simulink model "Radiometer_System_Model"  (R2019b)
settings: Solver=FixedStepDiscrete  StartTime=0.0  StopTime=0.00011  FixedStep=1/2500e6  RelTol=1e-3  EnableMultiTasking=on
values from neighbouring files (symbols this model uses):
  ADC_Clock = 2500e6    (= 2500000000)    [RunMe.m]
  divisionConst = 50    [RunMe.m]
libraries: dspsrcs4 x2
settings Model: Creator=tmacleod  LastModifiedBy=ian
settings SolverCC: AutoInsertRateTranBlk=on
settings DataIOCC: LimitDataPoints=on  SaveFormat=Array  ReturnWorkspaceOutputs=off
settings OptimizationCC: LifeSpan=inf
settings DebuggingCC: SolverPrmCheckMsg=warning  SFUnexpectedBacktrackingDiag=warning  SFNoUnconditionalDefaultTransitionDiag=warning  SFExecutionAtInitializationDiag=none  ArithmeticOperatorsInVariantConditions=warning
settings HardwareCC: ProdBitPerPointer=32  ProdBitPerSizeT=32  ProdBitPerPtrDiffT=32  ProdLargestAtomicFloat=None  ProdIntDivRoundTo=Undefined  ProdEndianess=Unspecified  ProdWordSize=32  ProdHWDeviceType=32-bit Generic
settings ModelReferenceCC: PropagateSignalLabelsOutOfModel=off
settings SFSimCC: SimUseLocalCustomCode=off  CustomCodeUndefinedFunction=UseInterfaceOnly
settings RTWCC: RTWUseLocalCustomCode=off
settings CodeAppCC: StateflowObjectComments=on
settings GRTTargetCC: TargetLangStandard=C89/C90 (ANSI)  GeneratePreprocessorConditionals=Disable all
settings ConfigComp: CovMetricSettings=dw  CovHtmlReporting=on  CovSaveCumulativeToWorkspaceVar=on  CovSaveSingleToWorkspaceVar=on  CovExternalEMLEnable=off  CovSFcnEnable=off

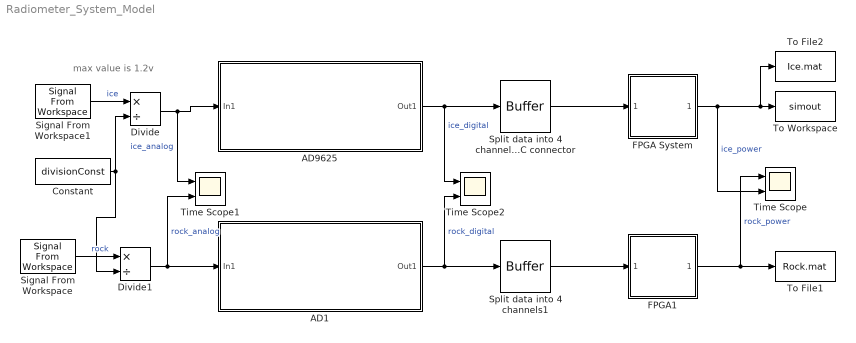
== system Radiometer_System_Model ==
  note: max value is 1.2v
  AD1 : Subsystem  mask{maskMode=ADC Only, maskDecimation=8, maskGain=0, maskNcoFreq=100e6, maskFclk=ADC_Clock, maskTessitura=147e6, maskExtJitter=60e-15, maskInputConfig=Absolute}
      mask prompts: maskMode "Mode of Operation"; maskDecimation "DDC Decimation"; maskGain "DDC Gain (dB)"; maskNcoFreq "NCO Frequency (Hz)"; maskFclk "Sampling Clock Frequency (Hz)"; maskTessitura "Mean Frequency (Hz)"; maskExtJitter "RMS Clock Jitter"; maskInputConfig "Input Configuration"
      mask init:
      | set_param([gcb '/AD9625 System Object'], 'Mode', maskMode);
      | set_param([gcb '/AD9625 System Object'], 'Decimation', maskDecimation);
      | set_param([gcb '/AD9625 System Object'], 'Gain', maskGain);
      | set_param([gcb '/AD9625 System Object'], 'NcoFreq', maskNcoFreq);
      | set_param([gcb '/AD9625 System Object'], 'Fclk', maskFclk);
      | set_param([gcb '/AD9625 System Object'], 'Tessitura', maskTessitura);
      | set_param([gcb '/AD9625 System Object'], 'ExtJitter', maskExtJitter);
      | set_param([gcb '/AD9625 System Object'], 'InputConfig', maskInputConfig);
      mask TypeOptions maskMode: ADC Only | ADC + DDC
      mask Callback maskMode:
      | % Get the mask parameter values. This is a cell
      | %   array of strings.
      | maskStr = get_param(gcb,'maskMode');
      | 
      | % The pop-up menu is the first mask parameter.
      | %   Check the value selected in the pop-up
      | if strcmp(maskStr,'ADC Only'),
      | 
      |     % Set the visibility of both parameters on when
      |     %   User-defined is selected in the pop-up.
      | 
      |     set_param(gcb,'MaskVisibilities',{'on';'off';'off';'off';'on';'on';'on';'on'}),
      | 
      | else
      | 
      |     % Turn off the visibility of the Value field
      |     %   when User-defined is not selected.
      | 
      |     set_param(gcb,'MaskVisibilities',{'on';'on';'on';'on';'on';'on';'on';'on'}),
      | 
      |     % Set the string in the Values field equal to the
      |     % string selected in the Gain pop-up menu.
      | 
      |     %maskStr{2}=maskStr{1};
      |     %set_param(gcb,'editvalue',maskStr);
      | end
      mask TypeOptions maskDecimation: 8 | 16
      mask TypeOptions maskGain: 0 | 6 | 12 | 18
      mask TypeOptions maskInputConfig: Normalized | Absolute
      mask Display:
      | port_label('input', 1, 'in (V)')
      | port_label('output', 1, 'out (Codes)')
  AD9625 : Subsystem  mask{maskMode=ADC Only, maskDecimation=8, maskGain=0, maskNcoFreq=100e6, maskFclk=ADC_Clock, maskTessitura=1e9, maskExtJitter=60e-15, maskInputConfig=Absolute}
      mask prompts: maskMode "Mode of Operation"; maskDecimation "DDC Decimation"; maskGain "DDC Gain (dB)"; maskNcoFreq "NCO Frequency (Hz)"; maskFclk "Sampling Clock Frequency (Hz)"; maskTessitura "Mean Frequency (Hz)"; maskExtJitter "RMS Clock Jitter"; maskInputConfig "Input Configuration"
      mask init: same as Radiometer_System_Model/AD1
      mask TypeOptions maskMode: ADC Only | ADC + DDC
      mask Callback maskMode:
      | % Get the mask parameter values. This is a cell
      | %   array of strings.
      | maskStr = get_param(gcb,'maskMode');
      | 
      | % The pop-up menu is the first mask parameter.
      | %   Check the value selected in the pop-up
      | if strcmp(maskStr,'ADC Only'),
      | 
      |     % Set the visibility of both parameters on when
      |     %   User-defined is selected in the pop-up.
      | 
      |     set_param(gcb,'MaskVisibilities',{'on';'off';'off';'off';'on';'on';'on';'on'}),
      | 
      | else
      | 
      |     % Turn off the visibility of the Value field
      |     %   when User-defined is not selected.
      | 
      |     set_param(gcb,'MaskVisibilities',{'on';'on';'on';'on';'on';'on';'on';'on'}),
      | 
      |     % Set the string in the Values field equal to the
      |     % string selected in the Gain pop-up menu.
      | 
      |     %maskStr{2}=maskStr{1};
      |     %set_param(gcb,'editvalue',maskStr);
      | end
      mask TypeOptions maskDecimation: 8 | 16
      mask TypeOptions maskGain: 0 | 6 | 12 | 18
      mask TypeOptions maskInputConfig: Normalized | Absolute
      mask Display:
      | port_label('input', 1, 'in (V)')
      | port_label('output', 1, 'out (Codes)')
  Constant : Constant  Value=divisionConst
  Divide : Product  Inputs=*/  SaturateOnIntegerOverflow=on  RndMeth=Zero
  Divide1 : Product  Inputs=*/  SaturateOnIntegerOverflow=on  RndMeth=Zero
  FPGA System : Subsystem  ReferencedSubsystem=FPGA
  FPGA1 : Subsystem  ReferencedSubsystem=FPGA
  Signal From Workspace : dspsrcs4/Signal From Workspace  X=vi_rockbase  Ts=1/ADC_Clock  nsamps=1  OutputAfterFinalValue=Setting to zero  ignoreOrWarnInputAndFrameLengths=off  OutputFrames=off
  Signal From Workspace1 : dspsrcs4/Signal From Workspace  X=vi_icebase  Ts=1/ADC_Clock  nsamps=1  OutputAfterFinalValue=Setting to zero  ignoreOrWarnInputAndFrameLengths=off  OutputFrames=off
  Split data into 4 channels modelling FMC connector : Buffer  N=4  OutputFrames=off
  Split data into 4 channels1 : Buffer  N=4  OutputFrames=off
  Time Scope : Scope  NumInputPorts=2
  Time Scope1 : Scope  NumInputPorts=2
  Time Scope2 : Scope  NumInputPorts=2
  To File1 : ToFile  Filename=Rock.mat  SaveFormat=Timeseries
  To File2 : ToFile  Filename=Ice.mat  SaveFormat=Timeseries
  To Workspace : ToWorkspace  VariableName=simout  SaveFormat=Timeseries  SampleTime=-1
  wires:
  AD9625/1(Out1) -> Time Scope2/1, Split data into 4 channels modelling FMC connector/1  "ice_digital"
  AD1/1(Out1) -> Time Scope2/2, Split data into 4 channels1/1  "rock_digital"
  Split data into 4 channels1/1 -> FPGA1/1
  FPGA1/1 -> Time Scope/1, To File1/1  "rock_power"
  FPGA System/1 -> To File2/1, To Workspace/1, Time Scope/2  "ice_power"
  Split data into 4 channels modelling FMC connector/1 -> FPGA System/1
  Divide/1 -> Time Scope1/1, AD9625/1(In1)  "ice_analog"
  Signal From Workspace1/1 -> Divide/1  "ice"
  Constant/1 -> Divide/2, Divide1/2
  Divide1/1 -> Time Scope1/2, AD1/1(In1)  "rock_analog"
  Signal From Workspace/1 -> Divide1/1  "rock"

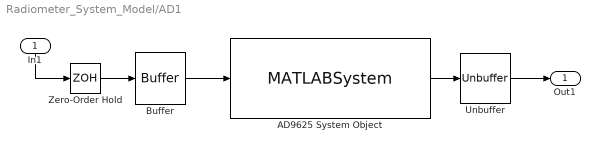
== system Radiometer_System_Model/AD1 ==
  In1 : Inport
  AD9625 System Object : MATLABSystem  System=AD9625_sysobj  Mode=ADC Only  Gain=0  NcoFreq=100e6  Fclk=ADC_Clock  Tessitura=147e6  ExtJitter=60e-15  InputConfig=Absolute  SimulateUsing=Interpreted execution
      settings: Decimation=8
      mask Type: AD9625_sysobj
      mask Display:
      | disp('AD9625');
      | port_label('input',1,'in (V)');
      | port_label('output',1,'out (Code)');
  Buffer : Buffer
  Unbuffer : Unbuffer
  Zero-Order Hold : ZeroOrderHold  SampleTime=1/2500e6
  Out1 : Outport
  wires:
  AD9625 System Object/1 -> Unbuffer/1
  In1/1 -> Zero-Order Hold/1
  Buffer/1 -> AD9625 System Object/1
  Zero-Order Hold/1 -> Buffer/1
  Unbuffer/1 -> Out1/1

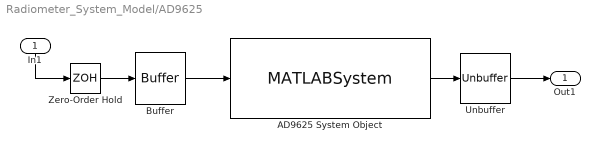
== system Radiometer_System_Model/AD9625 ==
  In1 : Inport
  AD9625 System Object : MATLABSystem  System=AD9625_sysobj  Mode=ADC Only  Gain=0  NcoFreq=100e6  Fclk=ADC_Clock  Tessitura=1e9  ExtJitter=60e-15  InputConfig=Absolute  SimulateUsing=Interpreted execution
      settings: Decimation=8
      mask Type: AD9625_sysobj
      mask Display:
      | disp('AD9625');
      | port_label('input',1,'in (V)');
      | port_label('output',1,'out (Code)');
  Buffer : Buffer
  Unbuffer : Unbuffer
  Zero-Order Hold : ZeroOrderHold  SampleTime=1/2500e6
  Out1 : Outport
  wires:
  AD9625 System Object/1 -> Unbuffer/1
  In1/1 -> Zero-Order Hold/1
  Buffer/1 -> AD9625 System Object/1
  Zero-Order Hold/1 -> Buffer/1
  Unbuffer/1 -> Out1/1
